simulink model "assign_r13"  (Simulink 5.0)
settings: Solver=ode45  StartTime=0.0  StopTime=110  RelTol=1e-3
libraries: simulink x1
CloseFcn:
  | rtwprivate ssgensfun ModelCloseRequest nlgentpl
settings Model: Creator=lbusoniu  LastModifiedBy=Administrator  ExtModeAutoUpdateStatusClock=off  BufferReuse=off  SaveTime=off  SaveOutput=off  OptimizeBlockIOStorage=off  RTWOptions="-aEnforceIntegerDowncast=1 -aFoldNonRolledExpr=1 -aInlineInvariantSignals=0 -aInlineParameters=0 -aLocalBlockOutputs=0 -aRollThreshold=5 -aGenerateReport=0 -aGenCodeOnly=0 -aRTWVerbose=1 -aIncludeHyperlinkInReport=0 -aLaunchReport=0 -aForceParamTrailComments=0 -aGenerateComments=1 -aIgnoreCustomStorageClasses=1 -aIncHierarchyInIds=0 -aMaxRTWIdLen=31 -aShowEliminatedStatements=0 -aPrefixModelToSubsysFcnNames=1 -aIncDataTypeInIds=0 -aInsertBlockDesc=0 -aSimulinkBlockComments=1 -aInlinedPrmAccess=\"Literals\"  -aSuppressErrorStatus=0 -aModelReferenceCompliant=1 -aSupportNonInlinedSFcns=1 -aSupportContinuousTime=1 -aSupportComplex=1 -aSupportNonFinite=1 -aSupportAbsoluteTime=1 -aTargetPreCompLibLocation=\"\" -aTargetLibSuffix=\"\" -aTargetFcnLib=\"ansi_tfl_tmw.mat\" -aMultiInstanceERTCode=0 -aLogVarNameModifier=\"rt_\" -aERTFirstTimeCompliant=0 -aIsPILTarget=0 -aCombineOutputUpdateFcns=0 -aGenerateASAP2=0 -aGenerateTestInterfaces=0 -aGenerateSampleERTMain=0 -aGenerateFullHeader=1 -aUtilityFuncGeneration=\"Auto\" -aIncludeFileDelimiter=\"Auto\" -aIncludeERTFirstTime=1 -aIncludeMdlTerminateFcn=1 -aPurelyIntegerCode=0 -aERTCustomFileBanners=0 -aRTWCAPIStates=0 -aRTWCAPIParams=0 -aRTWCAPISignals=0 -aMatFileLogging=1 -aGenFloatMathFcnCalls=\"ANSI_C\" -aExtModeMexFile=\"ext_comm\" -aExtModeTransport=0 -aExtModeStaticAllocSize=1000000 -aExtModeTesting=0 -aExtModeStaticAlloc=0 -aExtMode=0"

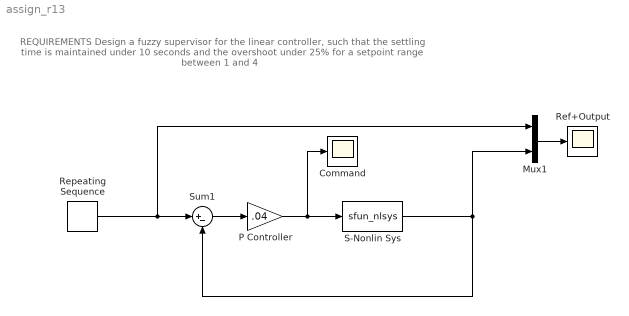
== system assign_r13 ==
  note: REQUIREMENTS
      | Design a fuzzy supervisor for the linear controller, such that
      | the settling time is maintained under 10 seconds and the overshoot under 25%
      | for a setpoint range between 1 and 4
  Command : Scope
      settings: TimeRange=120  YMin=-0.05  YMax=0.15  SaveName=u  DataFormat=Array
  Mux1 : Mux  Inputs=2
  P Controller : Gain  Gain=.04  SaturateOnIntegerOverflow=on
  Ref+Output : Scope
      settings: TimeRange=120  YMin=0  SaveName=u2  DataFormat=Array
  Repeating Sequence : simulink/Sources/Repeating Sequence  SystemSampleTime=-1  rep_seq_t=[0 15 15.5 30 30.5 45 45.5 60 60.5 75 75.5 90 91.5 111]  rep_seq_y=[1 1 .5 .5 2 2 1.5 1.5 3 3 2.5 2.5 4 4]
  S-Nonlin Sys : S-Function  FunctionName=sfun_nlsys
  Sum1 : Sum  Inputs=|+-  SaturateOnIntegerOverflow=on
  wires:
  Sum1/1 -> P Controller/1
  S-Nonlin Sys/1 -> Sum1/2, Mux1/2
  P Controller/1 -> S-Nonlin Sys/1, Command/1
  Mux1/1 -> Ref+Output/1
  Repeating Sequence/1 -> Sum1/1, Mux1/1
